simulink model "fin_3ph_2lvl"  (Simulink 7.5)
settings: Solver=ode45  StartTime=0.0  StopTime=0.1  RelTol=1e-3
undefined symbols (not defined in the file or in its folder): Ts
libraries: powerlib x38, powerlib_extras x1
settings Model: Creator=IS  LastModifiedBy=IS
settings SolverCC: ZeroCrossAlgorithm=Adaptive

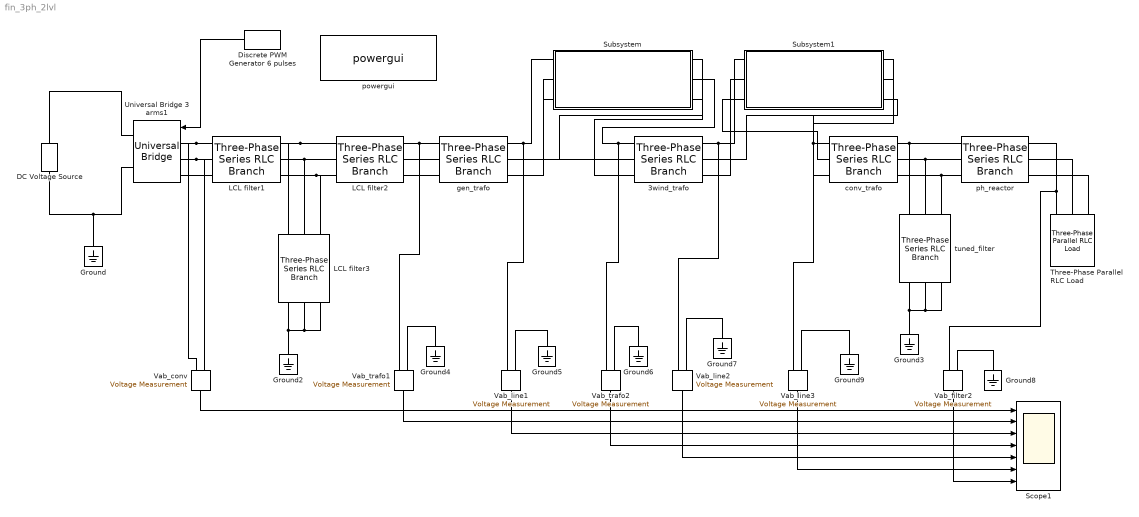
== system fin_3ph_2lvl ==
  3wind_trafo : powerlib/Elements/Three-Phase Series RLC Branch  DialogController=POWERSYS.PowerSysDialog  PhysicalDomain=powersysdomain  SubClassName=unknown  LeftPortType=p1  RightPortType=p1  LConnTagsString=A|B|C  RConnTagsString=A|B|C  BranchType=L  Resistance=1  Inductance=3.87e-2  Capacitance=1e-6  Measurements=None
  DC Voltage Source : powerlib/Electrical Sources/DC Voltage Source  DialogController=POWERSYS.PowerSysDialog  SystemSampleTime=-1  Amplitude=150e3  Measurements=None
  Discrete PWM Generator 6 pulses : powerlib_extras/Discrete  Control Blocks/Discrete PWM Generator  DialogController=POWERSYS.PowerSysDialog  SystemSampleTime=-1  GeneratorMode="3-arm  bridge (6 pulses)"  Fc=1080  Ts=Ts  Internal=on  mIndex=0.85  Freq=60  Phase=0
  Ground{,2..9} (9 alike) : powerlib/Elements/Ground  DialogController=POWERSYS.PowerSysDialog  PhysicalDomain=powersysdomain  SubClassName=unknown  LeftPortType=p1  RightPortType=p1  LConnTagsString=a
  LCL filter1 : powerlib/Elements/Three-Phase Series RLC Branch  DialogController=POWERSYS.PowerSysDialog  PhysicalDomain=powersysdomain  SubClassName=unknown  LeftPortType=p1  RightPortType=p1  LConnTagsString=A|B|C  RConnTagsString=A|B|C  BranchType=L  Resistance=1  Inductance=3.41e-3  Capacitance=1e-6  Measurements=None
  LCL filter2 : powerlib/Elements/Three-Phase Series RLC Branch  DialogController=POWERSYS.PowerSysDialog  PhysicalDomain=powersysdomain  SubClassName=unknown  LeftPortType=p1  RightPortType=p1  LConnTagsString=A|B|C  RConnTagsString=A|B|C  BranchType=L  Resistance=1  Inductance=1.82e-3  Capacitance=1e-6  Measurements=None
  LCL filter3 : powerlib/Elements/Three-Phase Series RLC Branch  DialogController=POWERSYS.PowerSysDialog  PhysicalDomain=powersysdomain  SubClassName=unknown  LeftPortType=p1  RightPortType=p1  LConnTagsString=A|B|C  RConnTagsString=A|B|C  BranchType=C  Resistance=1  Inductance=1e-3  Capacitance=5.24e-5  Measurements=None
  Scope1 : Scope  NumInputPorts=7
      settings: TimeRange=0.5  YMin=-500~-400~-5~-5~-5~-5~-5  YMax=500~500~5~5~5~5~5  SaveName=psb3phPWM1_str  MaxDataPoints=500000
  Subsystem : Subsystem
  Subsystem1 : Subsystem
  Three-Phase Parallel RLC Load : powerlib/Elements/Three-Phase Parallel RLC Load  DialogController=POWERSYS.PowerSysDialog  PhysicalDomain=powersysdomain  SubClassName=unknown  LeftPortType=p1  RightPortType=p1  LConnTagsString=A|B|C  Configuration=Y (grounded)  NominalVoltage=106e3  NominalFrequency=50  ActivePower=10e3  InductivePower=100  CapacitivePower=100  Measurements=None
  Universal Bridge 3 arms1 : powerlib/Power Electronics/Universal Bridge  DialogController=POWERSYS.PowerSysDialog  SystemSampleTime=-1  Arms=3  SnubberResistance=10000  SnubberCapacitance=inf  Device=IGBT / Diodes  Ron=1e-4  Lon=0  ForwardVoltages="[  1  1  ]"  ForwardVoltage=.8  GTOparameters=[ 10e-6 , 20e-6 ]  IGBTparameters=[ 1e-6 , 2e-6 ]  Measurements=None  Measurements_2=None  converterType=Rectifier
  Vab_conv : powerlib/Measurements/Voltage Measurement  Tag=PoWeRsYsTeMmEaSuReMeNt  DialogController=POWERSYS.PowerSysDialog  SystemSampleTime=-1  PhasorSimulation=off  OutputType=Magnitude  PSBequivalent=0
  Vab_filter2 : powerlib/Measurements/Voltage Measurement  Tag=PoWeRsYsTeMmEaSuReMeNt  DialogController=POWERSYS.PowerSysDialog  SystemSampleTime=-1  PhasorSimulation=off  OutputType=Magnitude  PSBequivalent=0
  Vab_line1 : powerlib/Measurements/Voltage Measurement  Tag=PoWeRsYsTeMmEaSuReMeNt  DialogController=POWERSYS.PowerSysDialog  SystemSampleTime=-1  PhasorSimulation=off  OutputType=Magnitude  PSBequivalent=0
  Vab_line2 : powerlib/Measurements/Voltage Measurement  Tag=PoWeRsYsTeMmEaSuReMeNt  DialogController=POWERSYS.PowerSysDialog  SystemSampleTime=-1  PhasorSimulation=off  OutputType=Magnitude  PSBequivalent=0
  Vab_line3 : powerlib/Measurements/Voltage Measurement  Tag=PoWeRsYsTeMmEaSuReMeNt  DialogController=POWERSYS.PowerSysDialog  SystemSampleTime=-1  PhasorSimulation=off  OutputType=Magnitude  PSBequivalent=0
  Vab_trafo1 : powerlib/Measurements/Voltage Measurement  Tag=PoWeRsYsTeMmEaSuReMeNt  DialogController=POWERSYS.PowerSysDialog  SystemSampleTime=-1  PhasorSimulation=off  OutputType=Magnitude  PSBequivalent=0
  Vab_trafo2 : powerlib/Measurements/Voltage Measurement  Tag=PoWeRsYsTeMmEaSuReMeNt  DialogController=POWERSYS.PowerSysDialog  SystemSampleTime=-1  PhasorSimulation=off  OutputType=Magnitude  PSBequivalent=0
  conv_trafo : powerlib/Elements/Three-Phase Series RLC Branch  DialogController=POWERSYS.PowerSysDialog  PhysicalDomain=powersysdomain  SubClassName=unknown  LeftPortType=p1  RightPortType=p1  LConnTagsString=A|B|C  RConnTagsString=A|B|C  BranchType=L  Resistance=1  Inductance=1.93e-2  Capacitance=1e-6  Measurements=None
  gen_trafo : powerlib/Elements/Three-Phase Series RLC Branch  DialogController=POWERSYS.PowerSysDialog  PhysicalDomain=powersysdomain  SubClassName=unknown  LeftPortType=p1  RightPortType=p1  LConnTagsString=A|B|C  RConnTagsString=A|B|C  BranchType=L  Resistance=1  Inductance=3.03e-3  Capacitance=1e-6  Measurements=None
  ph_reactor : powerlib/Elements/Three-Phase Series RLC Branch  DialogController=POWERSYS.PowerSysDialog  PhysicalDomain=powersysdomain  SubClassName=unknown  LeftPortType=p1  RightPortType=p1  LConnTagsString=A|B|C  RConnTagsString=A|B|C  BranchType=L  Resistance=1  Inductance=1.93e-2  Capacitance=1e-6  Measurements=None
  powergui : powerlib/powergui  Priority=1  SystemSampleTime=-1  SimulationMode=Continuous  SampleTime=50e-6  frequency=60  SPID=off  DisableSnubberDevices=off  DisableRonSwitches=off  DisableVfSwitches=off  SwTol=0  Interpol=off  frequencyindice=0  echomessages=off  HookPort=off  DisplayEquations=off  FunctionMessages=off  EnableUseOfTLC=off  x0status=blocks  RestoreLinks=warning  ResistiveCurrentMeasurement=off  Ylog=off  Xlog=on  ShowGrid=off  save=off  variable=ZData  structure=psb3phPWM1_str  ZoomFFT=off  StartTime=0.02  cycles=1  DisplayStyle=1  fundamental=50  FreqAxis=on  MaxFrequency=500  frequencyindicesteady=1  display=off  methode=off
  tuned_filter : powerlib/Elements/Three-Phase Series RLC Branch  DialogController=POWERSYS.PowerSysDialog  PhysicalDomain=powersysdomain  SubClassName=unknown  LeftPortType=p1  RightPortType=p1  LConnTagsString=A|B|C  RConnTagsString=A|B|C  BranchType=C  Resistance=1  Inductance=1e-3  Capacitance=5.66e-6  Measurements=None
  wires:
  Vab_filter2/1 -> Scope1/7
  Vab_line2/1 -> Scope1/5
  Vab_trafo2/1 -> Scope1/4
  Vab_line1/1 -> Scope1/3
  Vab_trafo1/1 -> Scope1/2
  Vab_conv/1 -> Scope1/1
  Discrete PWM Generator 6 pulses/1 -> Universal Bridge 3 arms1/1
  Vab_line3/1 -> Scope1/6
  connections:
  Universal Bridge 3 arms1/RConn1 -- DC Voltage Source/RConn1
  Universal Bridge 3 arms1/RConn2 -- DC Voltage Source/LConn1 -- Ground/LConn1
  Universal Bridge 3 arms1/LConn1 -- LCL filter1/LConn1 -- Vab_conv/LConn1
  LCL filter1/LConn2 -- Universal Bridge 3 arms1/LConn2 -- Vab_conv/LConn2
  Universal Bridge 3 arms1/LConn3 -- LCL filter1/LConn3
  LCL filter3/LConn1 -- LCL filter2/LConn1 -- LCL filter1/RConn1
  LCL filter3/LConn2 -- LCL filter1/RConn2 -- LCL filter2/LConn2
  LCL filter3/LConn3 -- LCL filter1/RConn3 -- LCL filter2/LConn3
  LCL filter3/RConn2 -- LCL filter3/RConn1 -- Ground2/LConn1 -- LCL filter3/RConn3
  LCL filter2/RConn1 -- gen_trafo/LConn1 -- Vab_trafo1/LConn1
  LCL filter2/RConn2 -- gen_trafo/LConn2
  LCL filter2/RConn3 -- gen_trafo/LConn3
  Subsystem/LConn1 -- gen_trafo/RConn1 -- Vab_line1/LConn1
  gen_trafo/RConn2 -- Subsystem/RConn1
  gen_trafo/RConn3 -- Subsystem/LConn2
  3wind_trafo/LConn1 -- Vab_trafo2/LConn1 -- Subsystem/RConn2
  Subsystem/LConn3 -- 3wind_trafo/LConn2
  Subsystem/RConn3 -- 3wind_trafo/LConn3
  Subsystem1/LConn1 -- 3wind_trafo/RConn1 -- Vab_line2/LConn1
  3wind_trafo/RConn2 -- Subsystem1/RConn1
  3wind_trafo/RConn3 -- Subsystem1/LConn2
  Subsystem1/RConn2 -- conv_trafo/LConn1 -- Vab_line3/LConn1
  tuned_filter/RConn1 -- Ground3/LConn1 -- tuned_filter/RConn2 -- tuned_filter/RConn3
  conv_trafo/RConn3 -- tuned_filter/LConn3 -- ph_reactor/LConn3
  conv_trafo/RConn2 -- tuned_filter/LConn2 -- ph_reactor/LConn2
  conv_trafo/RConn1 -- tuned_filter/LConn1 -- ph_reactor/LConn1
  Three-Phase Parallel RLC Load/LConn1 -- ph_reactor/RConn1 -- Vab_filter2/LConn1
  ph_reactor/RConn2 -- Three-Phase Parallel RLC Load/LConn2
  ph_reactor/RConn3 -- Three-Phase Parallel RLC Load/LConn3
  Vab_trafo1/LConn2 -- Ground4/LConn1
  Vab_line1/LConn2 -- Ground5/LConn1
  Vab_trafo2/LConn2 -- Ground6/LConn1
  Vab_line2/LConn2 -- Ground7/LConn1
  Vab_line3/LConn2 -- Ground9/LConn1
  Vab_filter2/LConn2 -- Ground8/LConn1
  conv_trafo/LConn2 -- Subsystem1/LConn3
  conv_trafo/LConn3 -- Subsystem1/RConn3

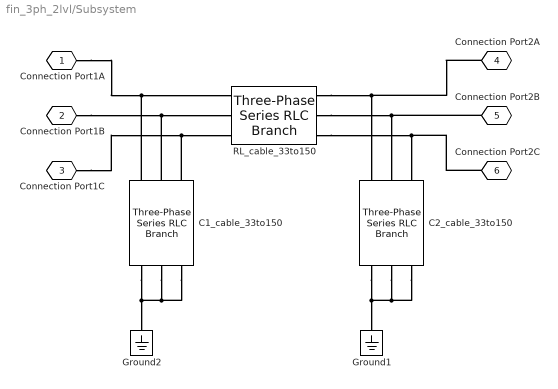
== system fin_3ph_2lvl/Subsystem ==
  C1_cable_33to150 : powerlib/Elements/Three-Phase Series RLC Branch  DialogController=POWERSYS.PowerSysDialog  PhysicalDomain=powersysdomain  SubClassName=unknown  LeftPortType=p1  RightPortType=p1  LConnTagsString=A|B|C  RConnTagsString=A|B|C  BranchType=C  Resistance=1  Inductance=1e-3  Capacitance=9.71e-4  Measurements=None
  C2_cable_33to150 : powerlib/Elements/Three-Phase Series RLC Branch  DialogController=POWERSYS.PowerSysDialog  PhysicalDomain=powersysdomain  SubClassName=unknown  LeftPortType=p1  RightPortType=p1  LConnTagsString=A|B|C  RConnTagsString=A|B|C  BranchType=C  Resistance=1  Inductance=1e-3  Capacitance=9.71e-4  Measurements=None
  Ground1 : powerlib/Elements/Ground  DialogController=POWERSYS.PowerSysDialog  PhysicalDomain=powersysdomain  SubClassName=unknown  LeftPortType=p1  RightPortType=p1  LConnTagsString=a
  Ground2 : powerlib/Elements/Ground  DialogController=POWERSYS.PowerSysDialog  PhysicalDomain=powersysdomain  SubClassName=unknown  LeftPortType=p1  RightPortType=p1  LConnTagsString=a
  RL_cable_33to150 : powerlib/Elements/Three-Phase Series RLC Branch  DialogController=POWERSYS.PowerSysDialog  PhysicalDomain=powersysdomain  SubClassName=unknown  LeftPortType=p1  RightPortType=p1  LConnTagsString=A|B|C  RConnTagsString=A|B|C  BranchType=RL  Resistance=2.19e-2  Inductance=1.07e-3  Capacitance=1e-6  Measurements=None
  Connection Port1A : PMIOPort  Tag=PMCPort  Port=1  Side=Left
  Connection Port1B : PMIOPort  Tag=PMCPort  Port=2  Side=Right
  Connection Port1C : PMIOPort  Tag=PMCPort  Port=3  Side=Left
  Connection Port2A : PMIOPort  Tag=PMCPort  Port=4  Side=Right
  Connection Port2B : PMIOPort  Tag=PMCPort  Port=5  Side=Left
  Connection Port2C : PMIOPort  Tag=PMCPort  Port=6  Side=Right
  connections:
  C2_cable_33to150/RConn2 -- Ground1/LConn1 -- C2_cable_33to150/RConn1 -- C2_cable_33to150/RConn3
  C1_cable_33to150/RConn2 -- Ground2/LConn1 -- C1_cable_33to150/RConn1 -- C1_cable_33to150/RConn3
  RL_cable_33to150/RConn1 -- C2_cable_33to150/LConn1 -- Connection Port2A/RConn1
  RL_cable_33to150/RConn2 -- C2_cable_33to150/LConn2 -- Connection Port2B/RConn1
  C1_cable_33to150/LConn2 -- RL_cable_33to150/LConn2 -- Connection Port1B/RConn1
  C1_cable_33to150/LConn3 -- RL_cable_33to150/LConn3 -- Connection Port1C/RConn1
  RL_cable_33to150/RConn3 -- C2_cable_33to150/LConn3 -- Connection Port2C/RConn1
  C1_cable_33to150/LConn1 -- RL_cable_33to150/LConn1 -- Connection Port1A/RConn1

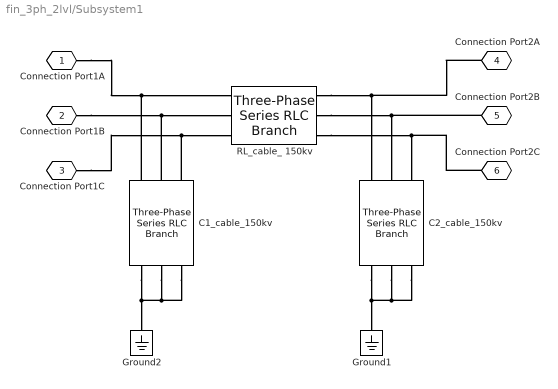
== system fin_3ph_2lvl/Subsystem1 ==
  C1_cable_150kv : powerlib/Elements/Three-Phase Series RLC Branch  DialogController=POWERSYS.PowerSysDialog  PhysicalDomain=powersysdomain  SubClassName=unknown  LeftPortType=p1  RightPortType=p1  LConnTagsString=A|B|C  RConnTagsString=A|B|C  BranchType=C  Resistance=1  Inductance=1e-3  Capacitance=5.2e-7  Measurements=None
  C2_cable_150kv : powerlib/Elements/Three-Phase Series RLC Branch  DialogController=POWERSYS.PowerSysDialog  PhysicalDomain=powersysdomain  SubClassName=unknown  LeftPortType=p1  RightPortType=p1  LConnTagsString=A|B|C  RConnTagsString=A|B|C  BranchType=C  Resistance=1  Inductance=1e-3  Capacitance=5.2e-7  Measurements=None
  Ground1 : powerlib/Elements/Ground  DialogController=POWERSYS.PowerSysDialog  PhysicalDomain=powersysdomain  SubClassName=unknown  LeftPortType=p1  RightPortType=p1  LConnTagsString=a
  Ground2 : powerlib/Elements/Ground  DialogController=POWERSYS.PowerSysDialog  PhysicalDomain=powersysdomain  SubClassName=unknown  LeftPortType=p1  RightPortType=p1  LConnTagsString=a
  RL_cable_ 150kv : powerlib/Elements/Three-Phase Series RLC Branch  DialogController=POWERSYS.PowerSysDialog  PhysicalDomain=powersysdomain  SubClassName=unknown  LeftPortType=p1  RightPortType=p1  LConnTagsString=A|B|C  RConnTagsString=A|B|C  BranchType=RL  Resistance=5.6e-2  Inductance=1e-3  Capacitance=1e-6  Measurements=None
  Connection Port1A : PMIOPort  Tag=PMCPort  Port=1  Side=Left
  Connection Port1B : PMIOPort  Tag=PMCPort  Port=2  Side=Right
  Connection Port1C : PMIOPort  Tag=PMCPort  Port=3  Side=Left
  Connection Port2A : PMIOPort  Tag=PMCPort  Port=4  Side=Right
  Connection Port2B : PMIOPort  Tag=PMCPort  Port=5  Side=Left
  Connection Port2C : PMIOPort  Tag=PMCPort  Port=6  Side=Right
  connections:
  C2_cable_150kv/RConn2 -- Ground1/LConn1 -- C2_cable_150kv/RConn1 -- C2_cable_150kv/RConn3
  C1_cable_150kv/RConn2 -- Ground2/LConn1 -- C1_cable_150kv/RConn1 -- C1_cable_150kv/RConn3
  RL_cable_ 150kv/RConn1 -- C2_cable_150kv/LConn1 -- Connection Port2A/RConn1
  RL_cable_ 150kv/RConn2 -- C2_cable_150kv/LConn2 -- Connection Port2B/RConn1
  C1_cable_150kv/LConn2 -- RL_cable_ 150kv/LConn2 -- Connection Port1B/RConn1
  C1_cable_150kv/LConn3 -- RL_cable_ 150kv/LConn3 -- Connection Port1C/RConn1
  RL_cable_ 150kv/RConn3 -- C2_cable_150kv/LConn3 -- Connection Port2C/RConn1
  C1_cable_150kv/LConn1 -- RL_cable_ 150kv/LConn1 -- Connection Port1A/RConn1
